simulink model "sldemo_lct_filter"  (Simulink 7.6)
settings: Solver=FixedStepDiscrete  StartTime=0.0  StopTime=10  RelTol=1e-3
PreLoadFcn:
  | FilterGain = single(0.7);
libraries: simulink x1
Description:
  | Inputs Passed by Value or Address
settings Model: Creator=The MathWorks Inc.  ExtModeAutoUpdateStatusClock=off
settings DataIOCC: SaveOutput=off  SaveTime=off
settings OptimizationCC: InlineParams=on  InlineInvariantSignals=on  ZeroExternalMemoryAtStartup=off  ZeroInternalMemoryAtStartup=off  InitFltsAndDblsToZero=on  OptimizeModelRefInitCode=on  LifeSpan=1
settings DebuggingCC: SaveWithParameterizedLinksMsg=none  SignalResolutionControl=TryResolveAllWithWarning  SolverPrmCheckMsg=none  MultiTaskDSMMsg=warning
settings HardwareCC: TargetUnknown=on
settings RTWCC: SystemTargetFile=ert.tlc  GenCodeOnly=on  TemplateMakefile=ert_default_tmf  Description=RTW Embedded Coder (no auto configuration)  GenerateReport=on  ProcessScript=ert_make_rtw_hook  IncludeHyperlinkInReport=on  LaunchReport=on  IncludeERTFirstTime=on
settings CodeAppCC: IgnoreCustomStorageClasses=off
settings ERTTargetCC: TargetFcnLib=ansi_tfl_tmw.mat  MultiwordLength=2048  GenerateSampleERTMain=on  IncludeMdlTerminateFcn=off  SuppressErrorStatus=on  InlinedParameterPlacement=NonHierarchical  ERTSrcFileBannerTemplate=example_banner.tlc  ERTHdrFileBannerTemplate=example_banner.tlc  ERTCustomFileTemplate=example_file_process.tlc  ConvertIfToSwitch=off

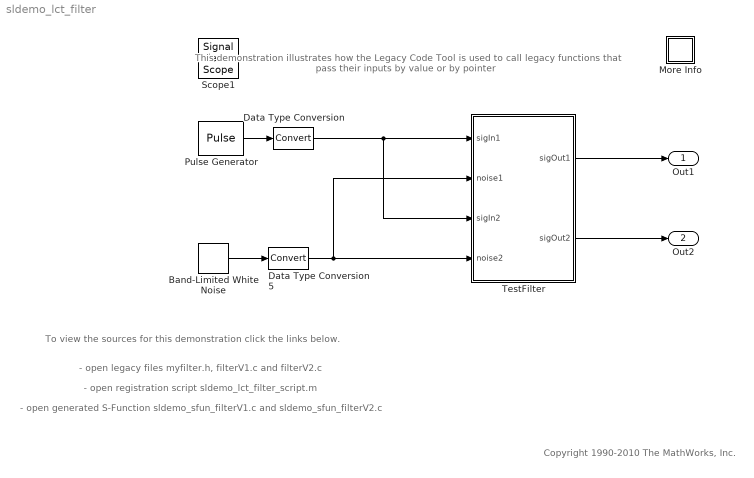
== system sldemo_lct_filter ==
  note: Copyright 1990-2010 The MathWorks, Inc.
  note: This demonstration illustrates how the Legacy Code Tool is used to
      | call legacy functions that pass their inputs by value or by pointer
  note: - open legacy files myfilter.h, filterV1.c and filterV2.c
  note: To view the sources for this demonstration
      | click the links below.
  note: - open registration script sldemo_lct_filter_script.m
  note: - open generated S-Function sldemo_sfun_filterV1.c and sldemo_sfun_filterV2.c
  Band-Limited White Noise : simulink/Sources/Band-Limited White Noise  SystemSampleTime=-1  Cov=[0.001]  Ts=0.1  seed=[23341]
  Data Type Conversion : DataTypeConversion  RndMeth=Zero
  Data Type Conversion5 : DataTypeConversion  RndMeth=Zero
  More Info : Subsystem
      settings: OpenFcn=showdemo('sldemo_lct_filter_script')
      mask Display: disp('?')
  Pulse Generator : DiscretePulseGenerator  Period=200  PulseWidth=100  PhaseDelay=10  SampleTime=0.1
  TestFilter : Subsystem
  Out1 : Outport
  Out2 : Outport  Port=2
  Scope1 : SignalViewerScope  IOType=viewer  NumInputPorts=2  RefreshTime=0.035000
      settings: YMin=-0.5~-0.5  YMax=1.5~1.5
  wires:
  Pulse Generator/1 -> Data Type Conversion/1
  Band-Limited White Noise/1 -> Data Type Conversion5/1
  TestFilter/1(sigOut1) -> Out1/1
  TestFilter/2(sigOut2) -> Out2/1
  Data Type Conversion/1 -> TestFilter/1(sigIn1), TestFilter/3(sigIn2)
  Data Type Conversion5/1 -> TestFilter/4(noise2), TestFilter/2(noise1)

== system sldemo_lct_filter/More Info ==

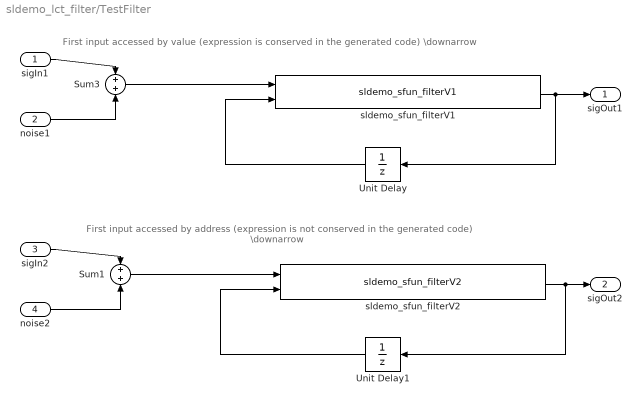
== system sldemo_lct_filter/TestFilter ==
  note: First input accessed by value
      |  (expression is conserved in the generated code)
      | \downarrow
  note: First input accessed by address
      |  (expression is not conserved in the generated code)
      | \downarrow
  sigIn1 : Inport
  noise1 : Inport  Port=2
  sigIn2 : Inport  Port=3
  noise2 : Inport  Port=4
  Sum1 : Sum
  Sum3 : Sum
  Unit Delay : UnitDelay  SampleTime=-1
  Unit Delay1 : UnitDelay  SampleTime=-1
  sldemo_sfun_filterV1 : S-Function  FunctionName=sldemo_sfun_filterV1  Parameters=SParameter1  EnableBusSupport=off  mask(Legacy Function){SFunctionSpec=single y1 = filterV1(single u1, single u2, single p1), SParameter1=FilterGain, ShowSpec=on}
      mask prompts: SParameter1 "P1:"; ShowSpec "Display function specification"
      mask help:
      | This block allows you to call the legacy functions specified by the following Legacy Code Tool definition:
      | def.SFunctionName = 'sldemo_sfun_filterV1';
      | def.OutputFcnSpec = 'single y1 = filterV1(single u1, single u2, single p1)';
      | def.HeaderFiles = {'myfilter.h'};
      | def.SourceFiles = {'filterV1.c'};
      | def.IncPaths = {'sldemo_lct_src'};
      | def.SrcPaths = {'sldemo_lct_src'};
      mask Help: <p>This block was generated automatically by the Legacy Code Tool. For detailed help on this tool, call<a href="matlab:legacy_code('help')"> legacy_code('help')</a>.</p>
      mask CallbackString:
      | ||if strcmp(get_param(gcbh, 'ShowSpec'), 'on')
      |   set_param(gcbh, 'MaskDisplay', sprintf('fprintf(''%s'');', get_param(gcbh, 'SFunctionSpec')));
      | else
      |   set_param(gcbh, 'MaskDisplay', sprintf('fprintf(''%s'');', get_param(gcbh, 'FunctionName')));
      | end
      mask Display: fprintf('single y1 = filterV1(single u1, single u2, single p1)');
  sldemo_sfun_filterV2 : S-Function  FunctionName=sldemo_sfun_filterV2  Parameters=SParameter1  EnableBusSupport=off  mask(Legacy Function){SFunctionSpec=single y1 = filterV2(single u1[1], single u2, single p1), SParameter1=FilterGain, ShowSpec=on}
      mask prompts: SParameter1 "P1:"; ShowSpec "Display function specification"
      mask help:
      | This block allows you to call the legacy functions specified by the following Legacy Code Tool definition:
      | def.SFunctionName = 'sldemo_sfun_filterV2';
      | def.OutputFcnSpec = 'single y1 = filterV2(single u1[1], single u2, single p1)';
      | def.HeaderFiles = {'myfilter.h'};
      | def.SourceFiles = {'filterV2.c'};
      | def.IncPaths = {'sldemo_lct_src'};
      | def.SrcPaths = {'sldemo_lct_src'};
      mask Help: <p>This block was generated automatically by the Legacy Code Tool. For detailed help on this tool, call<a href="matlab:legacy_code('help')"> legacy_code('help')</a>.</p>
      mask CallbackString:
      | ||if strcmp(get_param(gcbh, 'ShowSpec'), 'on')
      |   set_param(gcbh, 'MaskDisplay', sprintf('fprintf(''%s'');', get_param(gcbh, 'SFunctionSpec')));
      | else
      |   set_param(gcbh, 'MaskDisplay', sprintf('fprintf(''%s'');', get_param(gcbh, 'FunctionName')));
      | end
      mask Display: fprintf('single y1 = filterV2(single u1[1], single u2, single p1)');
  sigOut1 : Outport
  sigOut2 : Outport  Port=2
  wires:
  noise1/1 -> Sum3/2
  sldemo_sfun_filterV1/1 -> Unit Delay/1, sigOut1/1
  sldemo_sfun_filterV2/1 -> Unit Delay1/1, sigOut2/1
  sigIn1/1 -> Sum3/1
  noise2/1 -> Sum1/2
  sigIn2/1 -> Sum1/1
  Sum3/1 -> sldemo_sfun_filterV1/1
  Unit Delay/1 -> sldemo_sfun_filterV1/2
  Sum1/1 -> sldemo_sfun_filterV2/1
  Unit Delay1/1 -> sldemo_sfun_filterV2/2
